simulink model "project"  (R2018b)
settings: Solver=FixedStepAuto  StartTime=0.0  StopTime=1000  FixedStep=1  RelTol=1e-3
settings Model: Creator=computer  LastModifiedBy=computer
settings DebuggingCC: SignalResolutionControl=None

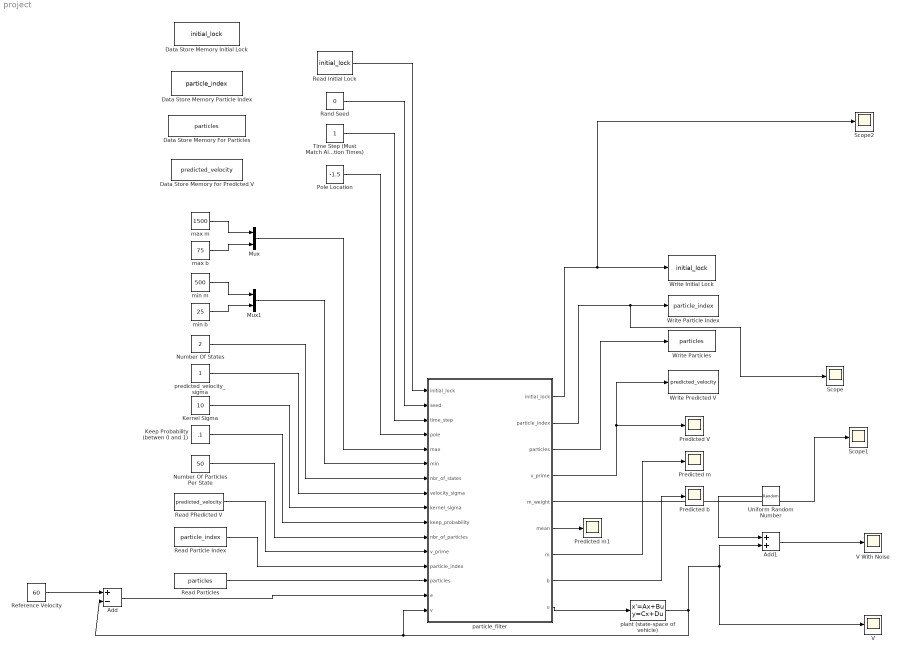
== system project ==
  Add : Sum  Inputs=+-
  Add1 : Sum
  Data Store Memory For Particles : DataStoreMemory  DataStoreName=particles  ReadBeforeWriteMsg=warning  WriteAfterWriteMsg=warning  WriteAfterReadMsg=warning  InitialValue=zeros(2, 50, 2)  ShowAdditionalParam=off  StateMustResolveToSignalObject=on
  Data Store Memory Initial Lock : DataStoreMemory  DataStoreName=initial_lock  ReadBeforeWriteMsg=warning  WriteAfterWriteMsg=warning  WriteAfterReadMsg=warning  ShowAdditionalParam=off
  Data Store Memory Particle Index : DataStoreMemory  DataStoreName=particle_index  ReadBeforeWriteMsg=warning  WriteAfterWriteMsg=warning  WriteAfterReadMsg=warning  ShowAdditionalParam=off
  Data Store Memory for Predicted V : DataStoreMemory  DataStoreName=predicted_velocity  ReadBeforeWriteMsg=warning  WriteAfterWriteMsg=warning  WriteAfterReadMsg=warning  ShowAdditionalParam=off
  Keep Probability (betwen 0 and 1) : Constant  Value=.1
  Kernel Sigma : Constant  Value=10
  Mux : Mux  Inputs=2
  Mux1 : Mux  Inputs=2
  Number Of Particles Per State : Constant  Value=50
  Number Of States : Constant  Value=2
  Pole Location : Constant  Value=-1.5
  Predicted V : Scope
  Predicted b : Scope
  Predicted m : Scope
  Predicted m1 : Scope
  Rand Seed : Constant  Value=0
  Read Initial Lock : DataStoreRead  DataStoreName=initial_lock
  Read PRedicted V : DataStoreRead  DataStoreName=predicted_velocity
  Read Particle Index : DataStoreRead  DataStoreName=particle_index
  Read Particles : DataStoreRead  DataStoreName=particles
  Reference Velocity : Constant  Value=60  SampleTime=1
  Scope : Scope
  Scope1 : Scope
  Scope2 : Scope
  Time Step (Must Match All Sample & Simulation Times) : Constant
  Uniform Random Number : UniformRandomNumber  Minimum=-10  Maximum=10  SampleTime=1
  V : Scope
  V With Noise : Scope
  Write Initial Lock : DataStoreWrite  DataStoreName=initial_lock
  Write Particle Index : DataStoreWrite  DataStoreName=particle_index
  Write Particles : DataStoreWrite  DataStoreName=particles
  Write Predicted V : DataStoreWrite  DataStoreName=predicted_velocity
  max b : Constant  Value=75
  max m : Constant  Value=1500
  min b : Constant  Value=25
  min m : Constant  Value=500
  particle_filter : MATLAB Function  TreatAsAtomicUnit=on
  plant (state-space of vehicle) : StateSpace  A=-50/1000  B=1/50  C=[1]  D=0  InitialCondition=0
  predicted_velocity_sigma : Constant
  wires:
  Uniform Random Number/1 -> Add1/1
  Reference Velocity/1 -> Add/1
  plant (state-space of vehicle)/1 -> Add1/2, V/1, particle_filter/16(v), Add/2
  Add1/1 -> V With Noise/1
  particle_filter/9(u) -> plant (state-space of vehicle)/1
  Add/1 -> particle_filter/15(e)
  Time Step (Must Match All Sample & Simulation Times)/1 -> particle_filter/3(time_step)
  Pole Location/1 -> particle_filter/4(pole)
  max m/1 -> Mux/1
  max b/1 -> Mux/2
  min b/1 -> Mux1/2
  min m/1 -> Mux1/1
  Mux/1 -> particle_filter/5(max)
  Mux1/1 -> particle_filter/6(min)
  Rand Seed/1 -> particle_filter/2(seed)
  Read Particles/1 -> particle_filter/14("particles ")
  particle_filter/3(particles) -> Write Particles/1
  Number Of States/1 -> particle_filter/7(nbr_of_states)
  Number Of Particles Per State/1 -> particle_filter/11(nbr_of_particles)
  Read Particle Index/1 -> particle_filter/13("particle_index ")
  particle_filter/2(particle_index) -> Scope/1, Write Particle Index/1
  Keep Probability (betwen 0 and 1)/1 -> particle_filter/10(keep_probability)
  particle_filter/4(v_prime) -> Write Predicted V/1, Predicted V/1
  Read PRedicted V/1 -> particle_filter/12("v_prime ")
  Kernel Sigma/1 -> particle_filter/9(kernel_sigma)
  predicted_velocity_sigma/1 -> particle_filter/8(velocity_sigma)
  Read Initial Lock/1 -> particle_filter/1("initial_lock ")
  particle_filter/1(initial_lock) -> Scope2/1, Write Initial Lock/1
  particle_filter/7(m) -> Predicted m/1
  particle_filter/8(b) -> Predicted b/1
  particle_filter/5(m_weight) -> Scope1/1
  particle_filter/6(mean) -> Predicted m1/1

== matlab function project/particle_filter ==
  settings: updateMethod=DISCRETE
  data: initial_lock output; initial_lock input; particle_index output; particles output; v_prime output; m_weight output; mean output; m output; b output; seed input; time_step input; pole input; max input; min input; nbr_of_states input; velocity_sigma input; kernel_sigma input; keep_probability input; nbr_of_particles input; v_prime input; particle_index input; particles input; e input; u output; v input
function [initial_lock, particle_index, particles, v_prime, m_weight, mean, m, b,u] = fcn(initial_lock,seed,time_step,pole,max,min,nbr_of_states,velocity_sigma,kernel_sigma,keep_probability,nbr_of_particles,v_prime,particle_index,particles,e,v)


% index particle
particle_index = particle_index + 1;

% update the particle weight
if ((initial_lock == 1) && (particle_index <= nbr_of_particles+1))
    particles = update_particle_weight(nbr_of_states,v_prime,v,particles,particle_index-1,velocity_sigma);
end


if(particle_index > nbr_of_particles)
    % resample particle
    particle_index = 1;
    particles = particle_resampler(particles, nbr_of_particles, keep_probability, kernel_sigma, nbr_of_states);
end



%% generate particles
% create particles initially
if (initial_lock == 0)
    particles = particle_generator(particles,nbr_of_states, nbr_of_particles, max, min, seed);
end

if (initial_lock == 0)
    initial_lock = 1;
end

%% sample particle
% preallocate array
particle = zeros([nbr_of_states, 1]);
test_weight = zeros([nbr_of_states, 1]);
test_mean = zeros([nbr_of_states, 1]);
if(particle_index <= nbr_of_particles)
    % return next particle
    for index = 1:nbr_of_states
        particle(index) = particles(index, particle_index, 1);
        test_weight(index) = particles(index, particle_index, 2);
        test_mean(index) = sum(particles(index, 1:nbr_of_particles, 1))/nbr_of_particles;
    end
end
m_weight = test_weight(1);
mean = test_mean(1);

%% utilize sample
% set particles equal to system
m = particle(1);
%b = particle(2);

b = 50;
%m = 1000;

%state-space matricies
A = [-b/m];
B = [1/b];
C = [1];
D = [0]; 

% controllability matrix
Pc = [B];

% Ackerman formula
K = [1]*inv(Pc)*(A+-pole);

% calculate next step
v_prime = v + time_step*(A*v+B*K*e);

% control law
u = K*e;
